simulink model "Main_Simulink"  (R2022b)
settings: Solver=ode4  StartTime=0.0  StopTime=3  FixedStep=0.01  MaxStep=0.01  MinStep=0.005  RelTol=1e-3  EnableMultiTasking=on
libraries: simulink_need_slupdate x1
settings Model: Creator=thora  LastModifiedBy=HP
settings SolverCC: ZeroCrossControl=DisableAll  ZeroCrossAlgorithm=Non-adaptive  AlgebraicLoopSolver=TrustRegion
settings DataIOCC: LimitDataPoints=on  SaveFormat=Array  SignalLoggingSaveFormat=ModelDataLogs  ReturnWorkspaceOutputs=off
settings OptimizationCC: ExpressionDepthLimit=2147483647  InitFltsAndDblsToZero=on  LifeSpan=inf
settings DebuggingCC: AlgebraicLoopMsg=none  UnderspecifiedInitializationDetection=Classic  MergeDetectMultiDrivingBlocksExec=none  SolverPrmCheckMsg=warning  FcnCallInpInsideContextMsg=warning  UnconnectedInputMsg=warning  UnconnectedOutputMsg=warning  UnconnectedLineMsg=warning  StateNameClashWarn=warning  SFUnexpectedBacktrackingDiag=warning  SFNoUnconditionalDefaultTransitionDiag=warning  SFExecutionAtInitializationDiag=none  SFMachineParentedDataDiag=warning  ArithmeticOperatorsInVariantConditions=warning
settings HardwareCC: ProdBitPerPointer=32  ProdBitPerSizeT=32  ProdBitPerPtrDiffT=32  ProdLargestAtomicFloat=None  ProdIntDivRoundTo=Undefined  ProdEndianess=Unspecified  ProdWordSize=32  ProdHWDeviceType=32-bit Generic
settings ModelReferenceCC: PropagateSignalLabelsOutOfModel=off
settings CodeAppCC: StateflowObjectComments=on
settings GRTTargetCC: TargetLangStandard=C89/C90 (ANSI)  CombineOutputUpdateFcns=off  GRTInterface=on
settings ConfigComp: CovMetricSettings=dw  CovSaveCumulativeToWorkspaceVar=on  CovSaveSingleToWorkspaceVar=on

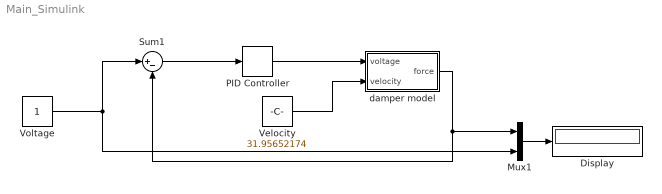
== system Main_Simulink ==
  Display : Display
  Mux1 : Mux  Inputs=2
  PID Controller : simulink_need_slupdate/PID Controller  P=1  I=1  D=1
  Sum1 : Sum  Inputs=|+-
  Velocity : Constant  Value=31.95652174
  Voltage : Constant
  damper model : Subsystem
  wires:
  Mux1/1 -> Display/1
  Sum1/1 -> PID Controller/1
  Voltage/1 -> Sum1/1, Mux1/2
  damper model/1(force) -> Sum1/2, Mux1/1
  PID Controller/1 -> damper model/1(voltage)
  Velocity/1 -> damper model/2(velocity)

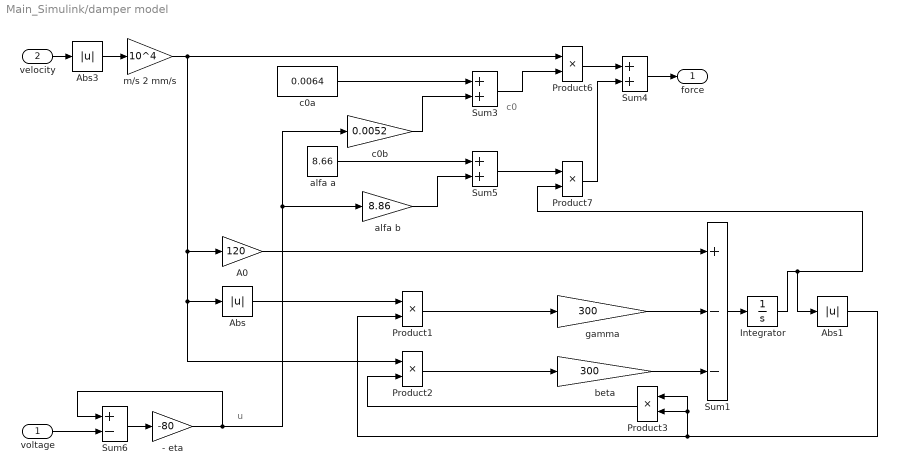
== system Main_Simulink/damper model ==
  note: c0
  note: u
  voltage : Inport
  velocity : Inport  Port=2
  - eta : Gain  Gain=-80  SaturateOnIntegerOverflow=on  OutDataTypeStr=Inherit: Same as input  ParamDataTypeStr=Inherit: Same as input
  A0 : Gain  Gain=120  SaturateOnIntegerOverflow=on  OutDataTypeStr=Inherit: Same as input  ParamDataTypeStr=Inherit: Same as input
  Abs : Abs  SaturateOnIntegerOverflow=off
  Abs1 : Abs  SaturateOnIntegerOverflow=off
  Abs3 : Abs
  Integrator : Integrator  LimitOutput=on  UpperSaturationLimit=0.01  LowerSaturationLimit=0
  Product{1..3,6..7} (5 alike) : Product  SaturateOnIntegerOverflow=on  OutDataTypeStr=Inherit: Same as first input
  Sum1 : Sum  Inputs=+--  SaturateOnIntegerOverflow=on
  Sum3 : Sum  SaturateOnIntegerOverflow=on
  Sum4 : Sum  SaturateOnIntegerOverflow=on
  Sum5 : Sum  SaturateOnIntegerOverflow=on
  Sum6 : Sum  Inputs=+-  SaturateOnIntegerOverflow=on
  alfa a : Constant  Value=8.66
  alfa b : Gain  Gain=8.86  SaturateOnIntegerOverflow=on  OutDataTypeStr=Inherit: Same as input  ParamDataTypeStr=Inherit: Same as input
  beta : Gain  Gain=300  SaturateOnIntegerOverflow=on  OutDataTypeStr=Inherit: Same as input  ParamDataTypeStr=Inherit: Same as input
  c0a : Constant  Value=0.0064
  c0b : Gain  Gain=0.0052  SaturateOnIntegerOverflow=on  OutDataTypeStr=Inherit: Same as input  ParamDataTypeStr=Inherit: Same as input
  gamma : Gain  Gain=300  SaturateOnIntegerOverflow=on  OutDataTypeStr=Inherit: Same as input  ParamDataTypeStr=Inherit: Same as input
  m/s 2 mm/s : Gain  Gain=10^4  SaturateOnIntegerOverflow=on  OutDataTypeStr=Inherit: Same as input  ParamDataTypeStr=Inherit: Same as input
  force : Outport
  wires:
  Sum4/1 -> force/1
  c0a/1 -> Sum3/1
  c0b/1 -> Sum3/2
  Sum3/1 -> Product6/2
  Product6/1 -> Sum4/1
  Product7/1 -> Sum4/2
  Sum5/1 -> Product7/1
  alfa a/1 -> Sum5/1
  alfa b/1 -> Sum5/2
  A0/1 -> Sum1/1
  Abs/1 -> Product1/1
  Product1/1 -> gamma/1
  Product2/1 -> beta/1
  Sum1/1 -> Integrator/1
  Integrator/1 -> Abs1/1, Product7/2
  Abs1/1 -> Product1/2, Product3/1, Product3/2
  Product3/1 -> Product2/2
  gamma/1 -> Sum1/2
  beta/1 -> Sum1/3
  m/s 2 mm/s/1 -> Product6/1, A0/1, Abs/1, Product2/1
  velocity/1 -> Abs3/1
  voltage/1 -> Sum6/2
  Sum6/1 -> - eta/1
  - eta/1 -> Sum6/1, c0b/1, alfa b/1
  Abs3/1 -> m/s 2 mm/s/1
